simulink model "svpwm_inv_Motor_new21b"  (R2021b)
settings: Solver=daessc  StartTime=0.0  StopTime=3.3  MaxStep=1e-6  RelTol=1e-3
libraries: fl_lib x30, nesl_utility x29, ee_lib x16, simulink x6, spsMeanLib x6, slpidlib x4, mcbcontrolslib x3, simulink_extras x1
(part 2 of 2)

== matlab function svpwm_inv_Motor_new21b/SVPWM ==
  data: vrefa input; vphase input; VDC input; IA input; IB input; Ts output
  events: trigger input RISING_EDGE_EVENT
%function [Ts1,Ts2,Ts3,Ts4,Ts5,Ts6] = fcn(vrefa,vphase,VDC,IA,IB)
function Ts   = fcn(vrefa,vphase,VDC,IA,IB)
%время 1/2 ШИМ периода
dt=100e-6;


%алгоритм формирования векторной ШИМ  мертвым веменем dead [мкс]
dead=1.0;
dead=dead/(dt*1e6);
a=vphase;
v2=vrefa*1.5;
if a>=0 && a<pi/3 
    n=1;
elseif  a>=pi/3 && a<2*pi/3 
    n=2;
elseif  a>=2*pi/3 && a<pi 
    n=3;
elseif  a>=pi && a<4*pi/3 
    n=4;
elseif  a>=4*pi/3 && a<5*pi/3 
    n=5;
else n=6;

end

a_cor=a-(n-1)*pi/3;

T1 = (v2/VDC)*sin(pi/3-a_cor)/sin(pi/3);
T2 = (v2/VDC)*sin(a_cor)/sin(pi/3);
T0=1-T1-T2;
Ta1=0; Ta3=0; Ta5=0; 
switch n
    case 1
        
        Ta1=T1+T2+T0/2;
        
        Ta3=T2+T0/2;
       
        Ta5=T0/2;
       
    case 2
        
        Ta1=T1+T0/2;
        
        Ta3=T1+T2+T0/2;
    
        Ta5=T0/2;       
        
    case 3
        
        Ta1=T0/2;
       
        Ta3=T1+T2+T0/2;
       
        Ta5=T2+T0/2;    
        
    case 4
        
        Ta1=T0/2;
       
        Ta3=T1+T0/2;
       
        Ta5=T1+T2+T0/2;   
       
    case 5
        
        Ta1=T2+T0/2;
        
        Ta3=T0/2;
        
        Ta5=T1+T2+T0/2;     
        
    case 6
        
        Ta1=T1+T2+T0/2;
        
        Ta3=T0/2;
     
        Ta5=T1+T0/2;    
        
end


Ts1=(Ta1)-dead/2; 
Ts3=(Ta3)-dead/2; 
Ts5=(Ta5)-dead/2;
Ts2=(Ta1)+dead/2; 
Ts4=(Ta3)+dead/2; 
Ts6=(Ta5)+dead/2;


%if (IA>0) 
%    Ts1=Ts1+dead/2;
%    Ts2=Ts2+dead/2;
%else
%    Ts1=Ts1-dead/2;
%    Ts2=Ts2-dead/2;           
%end
%if (IB>0) 
%    Ts3=Ts3+dead/2;
%    Ts4=Ts4+dead/2;
%else
%    Ts3=Ts3-dead/2;
%    Ts4=Ts4-dead/2; 
%end  
%if ((-IA-IB)>0) 
%    Ts5=Ts5+dead/2;
%    Ts6=Ts6+dead/2;
%else
%    Ts5=Ts5-dead/2;
%    Ts6=Ts6-dead/2;           
%end

Ts = [Ts1,Ts2,Ts3,Ts4,Ts5,Ts6];
return;
